simulink model "tether000Test1"  (R2022a)
settings: Solver=VariableStepAuto  StartTime=0.0  StopTime=duration_s  FixedStep=.1  RelTol=1e-3
values from neighbouring files (symbols this model uses):
  env = ENV.env    [tether000Test_ts.m]    (also in tether000_tsmc.m)
  tetherLength = totalUnstchLength    (= 200)    [tether000Test_ts.m]
  thr = OCT.tethers    [tether000Test_ts.m]    (also in tether000_tsmc.m)
undefined symbols (not defined in the file or in its folder): initializeVariantsFromBlock, tether000, tether000_cl, tethers, tethers_cl
libraries: nodeDragForce_ul x1, nodeNetBuoyForce_ul x1, nodeSpringDamperForce_ul x1, twoNodeTether_cl x1
settings Model: Creator=James Reed  LastModifiedBy=lhill8
settings SolverCC: AlgebraicLoopSolver=TrustRegion
settings DebuggingCC: UnconnectedInputMsg=warning  UnconnectedOutputMsg=warning  UnconnectedLineMsg=warning  SFMachineParentedDataDiag=warning  ArithmeticOperatorsInVariantConditions=warning
settings SFSimCC: CustomCodeUndefinedFunction=UseInterfaceOnly

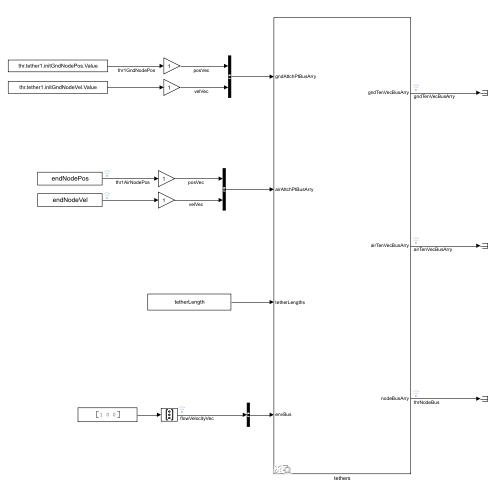
[thumbnail: Simulink's stored preview of the top-level diagram]
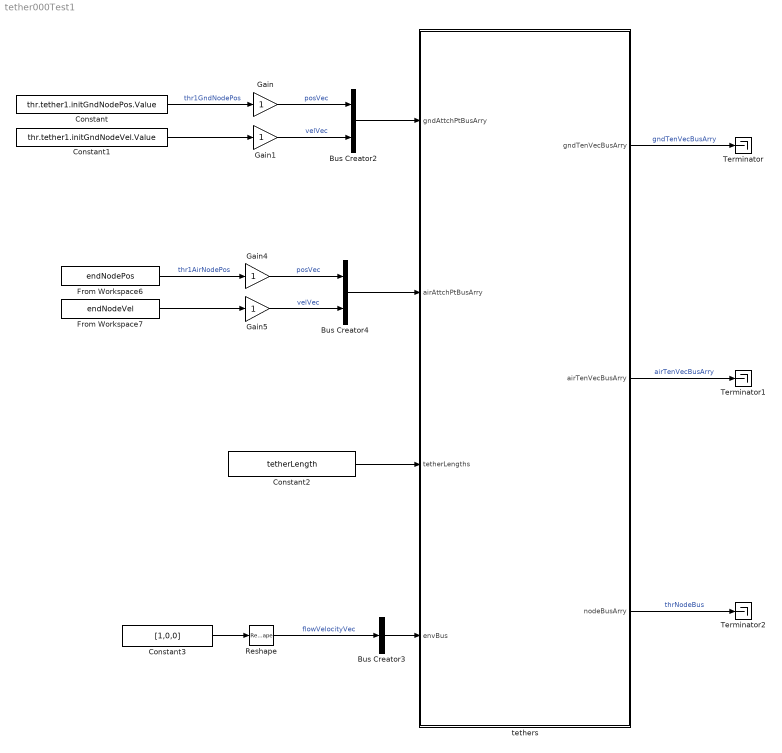
== system tether000Test1 ==
  Bus Creator2 : BusCreator  Inputs=2  OutDataTypeStr=Bus: thrAttachPtKinematicsBus  NonVirtualBus=on
  Bus Creator3 : BusCreator  Inputs=1  OutDataTypeStr=Bus:envBus
  Bus Creator4 : BusCreator  Inputs=2  OutDataTypeStr=Bus: thrAttachPtKinematicsBus  NonVirtualBus=on
  Constant : Constant  Value=thr.tether1.initGndNodePos.Value
  Constant1 : Constant  Value=thr.tether1.initGndNodeVel.Value
  Constant2 : Constant  Value=tetherLength
  Constant3 : Constant  Value=[1,0,0]
  From Workspace6 : FromWorkspace  VariableName=endNodePos
  From Workspace7 : FromWorkspace  VariableName=endNodeVel
  Gain{,1,4..5} (4 alike) : Gain
  Reshape : Reshape  OutputDimensionality=Column vector (2-D)
  Terminator : Terminator
  Terminator1 : Terminator
  Terminator2 : Terminator
  tethers : Subsystem  AncestorBlock=tethers_cl/tethers  LoadFcn=initializeVariantsFromBlock(gcb)  InitFcn=initializeVariantsFromBlock(gcb)  StartFcn=initializeVariantsFromBlock(gcb)  Variant=on
      settings: PreSaveFcn=initializeVariantsFromBlock(gcb)
  wires:
  Gain4/1 -> Bus Creator4/1  "posVec"
  From Workspace7/1 -> Gain5/1
  Gain5/1 -> Bus Creator4/2  "velVec"
  Constant1/1 -> Gain1/1
  Bus Creator3/1 -> tethers/4(envBus)
  Gain1/1 -> Bus Creator2/2  "velVec"
  tethers/3(nodeBusArry) -> Terminator2/1  "thrNodeBus"
  Constant/1 -> Gain/1  "thr1GndNodePos"
  Gain/1 -> Bus Creator2/1  "posVec"
  tethers/2(airTenVecBusArry) -> Terminator1/1  "airTenVecBusArry"
  Constant3/1 -> Reshape/1
  Reshape/1 -> Bus Creator3/1  "flowVelocityVec"
  Bus Creator2/1 -> tethers/1(gndAttchPtBusArry)
  From Workspace6/1 -> Gain4/1  "thr1AirNodePos"
  Constant2/1 -> tethers/3(tetherLengths)
  Bus Creator4/1 -> tethers/2(airAttchPtBusArry)
  tethers/1(gndTenVecBusArry) -> Terminator/1  "gndTenVecBusArry"

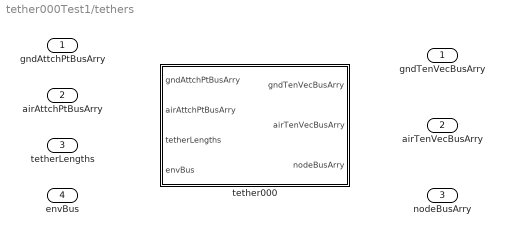
== system tether000Test1/tethers ==
  gndAttchPtBusArry : Inport
  airAttchPtBusArry : Inport  Port=2
  tetherLengths : Inport  Port=3
  envBus : Inport  Port=4  OutDataTypeStr=Bus: envBus
  tether000 : Subsystem  AncestorBlock=tether000_cl/tether000  InitFcn=tether000_init  Variant=on  VariantControl=VSS_tethers_tether000  mask{numNodes=thr.numNodes.Value, thrStructure=thr.struct('OCT.tether'), fluidDensity=env.water.density.Value, gravity=env.gravAccel.Value}
      mask prompts: numNodes "Num Nodes"; thrStructure "Tether Structure"; fluidDensity "Fluid Density"; gravity "Gravitational Acceleration"
  gndTenVecBusArry : Outport  VectorParamsAs1DForOutWhenUnconnected=off
  airTenVecBusArry : Outport  Port=2  VectorParamsAs1DForOutWhenUnconnected=off
  nodeBusArry : Outport  Port=3  VectorParamsAs1DForOutWhenUnconnected=off

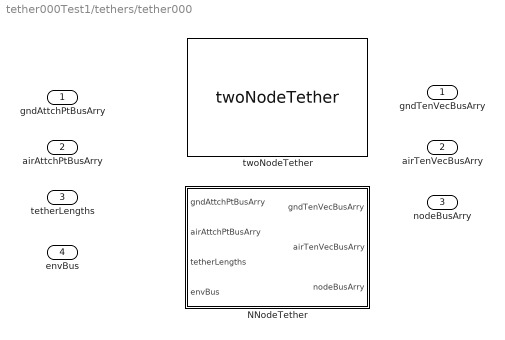
== system tether000Test1/tethers/tether000 ==
  gndAttchPtBusArry : Inport  OutDataTypeStr=Bus: thrAttachPtKinematicsBus
  airAttchPtBusArry : Inport  Port=2  OutDataTypeStr=Bus: thrAttachPtKinematicsBus
  tetherLengths : Inport  Port=3
  envBus : Inport  Port=4  OutDataTypeStr=Bus: envBus
  NNodeTether : Subsystem  AncestorBlock=NNodeTether_cl/NNodeTether/NNodeTether  VariantControl=numNodes~=2  mask{thr=thrStructure, flowDensity=fluidDensity, gravity=gravity}
      mask prompts: thr "Tether Structure"; flowDensity "Fluid Density"; gravity "Gravitational Acceleration"
  twoNodeTether : twoNodeTether_cl/twoNodeTether  VariantControl=numNodes==2  thr=thrStructure  flowDensity=fluidDensity  gravity=gravity
  gndTenVecBusArry : Outport  VectorParamsAs1DForOutWhenUnconnected=off
  airTenVecBusArry : Outport  Port=2  VectorParamsAs1DForOutWhenUnconnected=off
  nodeBusArry : Outport  Port=3  VectorParamsAs1DForOutWhenUnconnected=off

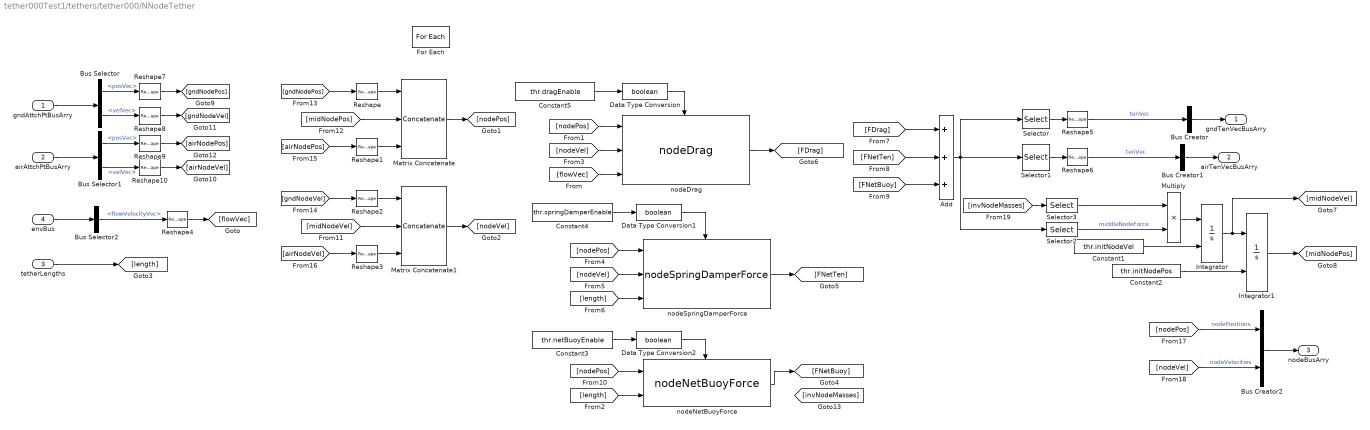
== system tether000Test1/tethers/tether000/NNodeTether ==
  gndAttchPtBusArry : Inport  OutDataTypeStr=Bus: thrAttachPtKinematicsBus  Partition=on  PartitionDimension=1  PartitionWidth=1  PartitionOffset=0
  airAttchPtBusArry : Inport  Port=2  OutDataTypeStr=Bus: thrAttachPtKinematicsBus  Partition=on  PartitionDimension=1  PartitionWidth=1  PartitionOffset=0
  tetherLengths : Inport  Port=3  Partition=on  PartitionDimension=1  PartitionWidth=1  PartitionOffset=0
  envBus : Inport  Port=4  OutDataTypeStr=Bus: envBus
  Add : Sum  Inputs=3
  Bus Creator : BusCreator  Inputs=1  OutDataTypeStr=Bus: thrTenVecBus  NonVirtualBus=on
  Bus Creator1 : BusCreator  Inputs=1  OutDataTypeStr=Bus: thrTenVecBus  NonVirtualBus=on
  Bus Creator2 : BusCreator  Inputs=2  OutDataTypeStr=Bus: thrNodeBus  NonVirtualBus=on
  Bus Selector : BusSelector  OutputSignals=posVec,velVec
  Bus Selector1 : BusSelector  OutputSignals=posVec,velVec
  Bus Selector2 : BusSelector  OutputSignals=flowVelocityVec
  Constant1 : Constant  Value=thr.initNodeVel
  Constant2 : Constant  Value=thr.initNodePos
  Constant3 : Constant  Value=thr.netBuoyEnable
  Constant4 : Constant  Value=thr.springDamperEnable
  Constant5 : Constant  Value=thr.dragEnable
  Data Type Conversion : DataTypeConversion  OutDataTypeStr=boolean  SaturateOnIntegerOverflow=off  RndMeth=Floor
  Data Type Conversion1 : DataTypeConversion  OutDataTypeStr=boolean  SaturateOnIntegerOverflow=off  RndMeth=Floor
  Data Type Conversion2 : DataTypeConversion  OutDataTypeStr=boolean  SaturateOnIntegerOverflow=off  RndMeth=Floor
  For Each : ForEach  DisableCoverage=on  IterateSubsysMaskParameter=on,off,off  SubsysMaskParameterIterationDimension=2,1,1  SubsysMaskParameterIterationStepSize=1,1,1
  Integrator : Integrator  InitialConditionSource=external
  Integrator1 : Integrator  InitialConditionSource=external
  Matrix Concatenate : Concatenate  NumInputs=3  Mode=Multidimensional array  ConcatenateDimension=2
  Matrix Concatenate1 : Concatenate  NumInputs=3  Mode=Multidimensional array  ConcatenateDimension=2
  Multiply : Product
  Reshape{,1..10} (11 alike) : Reshape  OutputDimensionality=Column vector (2-D)
  Selector : Selector  NumberOfDimensions=2  InputPortWidth=3  IndexOptions=Select all,Index vector (dialog)  Indices=[1 3],1  OutputSizes=1,1
  Selector1 : Selector  NumberOfDimensions=2  InputPortWidth=3  IndexOptions=Select all,Starting index (dialog)  Indices=[1 3],numNodes  OutputSizes=1,1
  Selector2 : Selector  NumberOfDimensions=2  InputPortWidth=3  IndexOptions=Select all,Index vector (dialog)  Indices=[1 3],2:numNodes-1  OutputSizes=1,1
  Selector3 : Selector  NumberOfDimensions=2  InputPortWidth=3  IndexOptions=Select all,Index vector (dialog)  Indices=[1 3],2:numNodes-1  OutputSizes=1,1
  nodeDrag : nodeDragForce_ul/nodeDrag  flowDensity=flowDensity  thrDiam=thr.diameter  dragCoeff=thr.dragCoeff
  nodeNetBuoyForce : nodeNetBuoyForce_ul/nodeNetBuoyForce  fluidDensity=flowDensity  tetherDensity=thr.density  diameter=thr.diameter  gravity=gravity
  nodeSpringDamperForce : nodeSpringDamperForce_ul/nodeSpringDamperForce  mass=thr.vehicleMass  zeta=thr.dampingRatio  diameter=thr.diameter  youngsMod=thr.youngsMod
  gndTenVecBusArry : Outport  ConcatenationDimension=1  VectorParamsAs1DForOutWhenUnconnected=off
  airTenVecBusArry : Outport  Port=2  ConcatenationDimension=1  VectorParamsAs1DForOutWhenUnconnected=off
  nodeBusArry : Outport  Port=3  ConcatenationDimension=1  VectorParamsAs1DForOutWhenUnconnected=off
  wires:
  Matrix Concatenate1/1 -> [nodeVel]
  [invNodeMasses] -> Selector3/1
  Selector3/1 -> Multiply/1
  Constant2/1 -> Integrator1/2
  Constant1/1 -> Integrator/2
  Data Type Conversion/1 -> nodeDrag/Enable
  Constant5/1 -> Data Type Conversion/1
  Data Type Conversion1/1 -> nodeSpringDamperForce/Enable
  Constant4/1 -> Data Type Conversion1/1
  Constant3/1 -> Data Type Conversion2/1
  Data Type Conversion2/1 -> nodeNetBuoyForce/Enable
  Multiply/1 -> Integrator/1
  [nodePos] -> Bus Creator2/1  "nodePositions"
  Reshape5/1 -> Bus Creator/1  "tenVec"
  Reshape6/1 -> Bus Creator1/1  "tenVec"
  Bus Creator1/1 -> airTenVecBusArry/1
  [nodeVel] -> Bus Creator2/2  "nodeVelocities"
  Bus Creator/1 -> gndTenVecBusArry/1
  Bus Creator2/1 -> nodeBusArry/1
  Reshape4/1 -> [flowVec]
  Reshape8/1 -> [gndNodeVel]
  Bus Selector/1 -> Reshape7/1  "<posVec>"
  Bus Selector1/2 -> Reshape10/1  "<velVec>"
  Reshape7/1 -> [gndNodePos]
  Bus Selector2/1 -> Reshape4/1  "<flowVelocityVec>"
  Reshape9/1 -> [airNodePos]
  Bus Selector1/1 -> Reshape9/1  "<posVec>"
  tetherLengths/1 -> [length]
  gndAttchPtBusArry/1 -> Bus Selector/1
  envBus/1 -> Bus Selector2/1
  Bus Selector/2 -> Reshape8/1  "<velVec>"
  airAttchPtBusArry/1 -> Bus Selector1/1
  Reshape10/1 -> [airNodeVel]
  Matrix Concatenate/1 -> [nodePos]
  [midNodePos] -> Matrix Concatenate/2
  [midNodeVel] -> Matrix Concatenate1/2
  Integrator1/1 -> [midNodePos]
  Integrator/1 -> Integrator1/1, [midNodeVel]
  Selector2/1 -> Multiply/2  "middleNodeForce"
  [gndNodePos] -> Reshape/1
  [gndNodeVel] -> Reshape2/1
  [airNodePos] -> Reshape1/1
  [airNodeVel] -> Reshape3/1
  Reshape/1 -> Matrix Concatenate/1
  Reshape1/1 -> Matrix Concatenate/3
  Reshape3/1 -> Matrix Concatenate1/3
  Reshape2/1 -> Matrix Concatenate1/1
  [flowVec] -> nodeDrag/3
  [nodePos] -> nodeDrag/1
  [length] -> nodeNetBuoyForce/2
  [nodeVel] -> nodeDrag/2
  [nodeVel] -> nodeSpringDamperForce/2
  [nodePos] -> nodeSpringDamperForce/1
  [length] -> nodeSpringDamperForce/3
  ? -> [invNodeMasses]
  nodeNetBuoyForce/1 -> [FNetBuoy]
  nodeSpringDamperForce/1 -> [FNetTen]
  nodeDrag/1 -> [FDrag]
  [FNetTen] -> Add/2
  [FDrag] -> Add/1
  [FNetBuoy] -> Add/3
  Selector/1 -> Reshape5/1
  Add/1 -> Selector/1, Selector2/1, Selector1/1
  Selector1/1 -> Reshape6/1
  [nodePos] -> nodeNetBuoyForce/1
